simulink model "LW7Q3"  (R2020b)
settings: Solver=VariableStepAuto  StartTime=0.0  StopTime=31  RelTol=1e-3
libraries: simulink_extras x7, dspsrcs4 x1
settings Model: Creator=Andy  LastModifiedBy=Andy

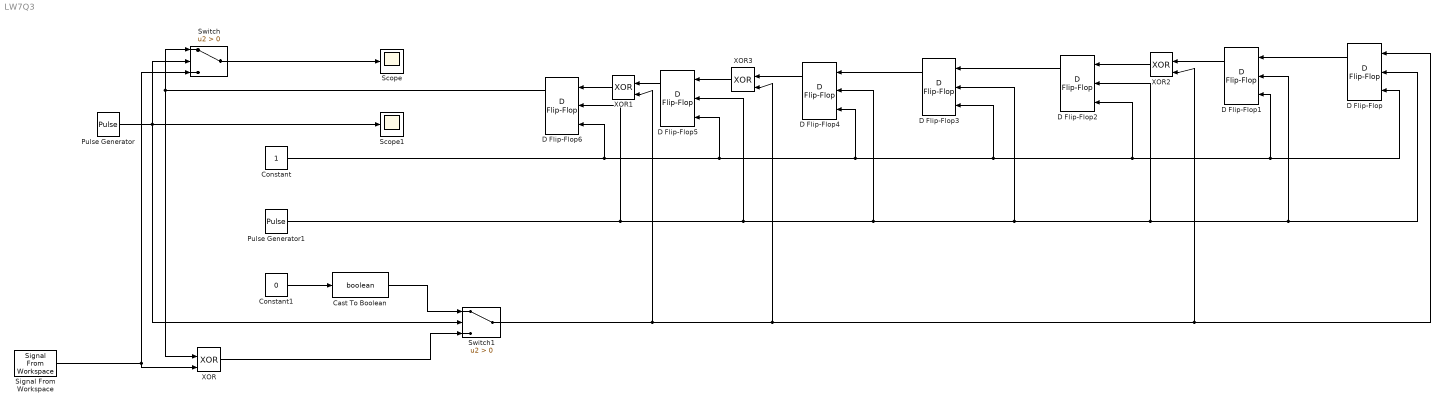
== system LW7Q3 ==
  Cast To Boolean : DataTypeConversion  OutDataTypeStr=boolean
  Constant : Constant
  Constant1 : Constant  Value=0
  D Flip-Flop{,1..6} (7 alike) : simulink_extras/Flip Flops/D Flip-Flop
  Pulse Generator : DiscretePulseGenerator  PulseType=Time based  Period=31  PulseWidth=25  PhaseDelay=24
  Pulse Generator1 : DiscretePulseGenerator  PulseType=Time based  Period=1  PulseWidth=50
  Scope : Scope
  Scope1 : Scope
  Signal From Workspace : dspsrcs4/Signal From Workspace  X=[0 1 0 1 0 1 0 0 0 1 0 1 0 0 1 0 0 1 0 0 1 1 1 0 0 0 0 0 0 0 0]  Ts=1  nsamps=1  OutputAfterFinalValue=Setting to zero  ignoreOrWarnInputAndFrameLengths=off  OutputFrames=off
  Switch : Switch  Criteria=u2 > Threshold
  Switch1 : Switch  Criteria=u2 > Threshold
  XOR{,1..3} (4 alike) : Logic  Operator=XOR  IconShape=distinctive  AllPortsSameDT=off  OutDataTypeStr=boolean
  wires:
  D Flip-Flop2/1 -> D Flip-Flop3/1
  XOR3/1 -> D Flip-Flop5/1
  XOR/1 -> Switch1/3
  Signal From Workspace/1 -> Switch/3, XOR/2
  Constant/1 -> D Flip-Flop4/3, D Flip-Flop3/3, D Flip-Flop2/3, D Flip-Flop1/3, D Flip-Flop/3, D Flip-Flop5/3, D Flip-Flop6/3
  Switch1/1 -> XOR1/2, XOR2/2, D Flip-Flop/1, XOR3/2
  Constant1/1 -> Cast To Boolean/1
  D Flip-Flop1/1 -> XOR2/1
  Pulse Generator1/1 -> D Flip-Flop4/2, D Flip-Flop3/2, D Flip-Flop2/2, D Flip-Flop1/2, D Flip-Flop/2, D Flip-Flop5/2, D Flip-Flop6/2
  D Flip-Flop3/1 -> D Flip-Flop4/1
  Switch/1 -> Scope/1
  Cast To Boolean/1 -> Switch1/1
  XOR2/1 -> D Flip-Flop2/1
  D Flip-Flop4/1 -> XOR3/1
  D Flip-Flop6/1 -> Switch/1, XOR/1
  Pulse Generator/1 -> Switch1/2, Switch/2, Scope1/1
  D Flip-Flop/1 -> D Flip-Flop1/1
  D Flip-Flop5/1 -> XOR1/1
  XOR1/1 -> D Flip-Flop6/1
